simulink model "doc_agc_compare_rectifier_and_square_law"  (R2014a)
settings: Solver=FixedStepDiscrete  StartTime=0.0  StopTime=300  RelTol=1e-3
libraries: commrfcorlib x2, commdigbbndpm3 x1, commrandsrc2 x1
settings Model: Creator=The MathWorks Inc.
settings DebuggingCC: UnderspecifiedInitializationDetection=Classic  StateNameClashWarn=warning

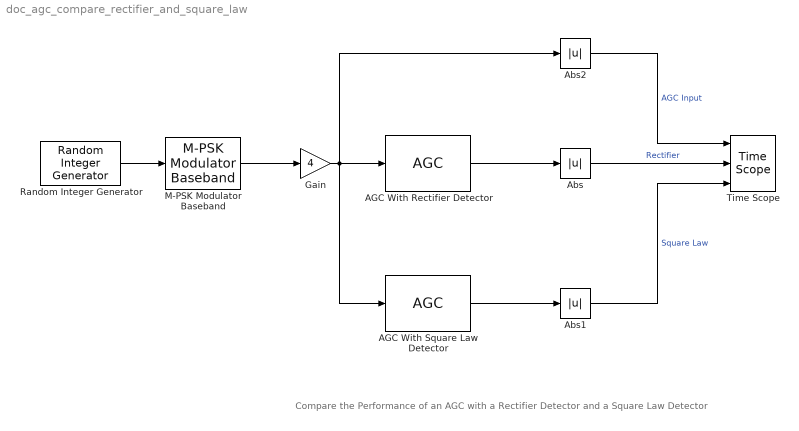
== system doc_agc_compare_rectifier_and_square_law ==
  note: Compare the Performance of an AGC with a Rectifier Detector and a Square Law Detector
  AGC With Rectifier Detector : commrfcorlib/AGC  SimulateUsing=Code generation  DetectorMethod=Rectifier  LoopMethod=Linear  UpdatePeriod=10  StepSize=0.1  MaximumGain=30  GainOutputPort=off
  AGC With Square Law Detector : commrfcorlib/AGC  SimulateUsing=Code generation  DetectorMethod=Square Law  LoopMethod=Linear  UpdatePeriod=10  StepSize=0.1  MaximumGain=30  GainOutputPort=off
  Abs : Abs
  Abs1 : Abs
  Abs2 : Abs
  Gain : Gain  Gain=4
  M-PSK Modulator Baseband : commdigbbndpm3/M-PSK Modulator Baseband  M=4  InType=Integer  Enc=Gray  Mapping=[0:7]  Ph=pi/4  outDtype=double  outWordLen=16  outUDDataType=sfix(16)  outFracLenMode=Best precision  outFracLen=15
  Random Integer Generator : commrandsrc2/Random Integer Generator  mul=4  seed=37  Ts=1  frameBased=on  sampPerFrame=100  orient=off  outDataType=double
  Time Scope : TimeScope  NumInputPorts=3  DefaultConfigurationName=spbscopes.TimeScopeBlockCfg
  wires:
  Random Integer Generator/1 -> M-PSK Modulator Baseband/1
  M-PSK Modulator Baseband/1 -> Gain/1
  AGC With Rectifier Detector/1 -> Abs/1
  Gain/1 -> Abs2/1, AGC With Square Law Detector/1, AGC With Rectifier Detector/1
  AGC With Square Law Detector/1 -> Abs1/1
  Abs/1 -> Time Scope/2  "Rectifier"
  Abs1/1 -> Time Scope/3  "Square Law"
  Abs2/1 -> Time Scope/1  "AGC Input"
